simulink model "Test2Part4a"  (R2024a)
settings: Solver=FixedStepAuto  StartTime=0  StopTime=1000  FixedStep=1  MaxStep=1  MinStep=1  RelTol=1e-3
libraries: matrix_library x2
settings Model: NumberOfSteps=1000  Creator=katutu  LastModifiedBy=katutu
settings HardwareCC: ProdBitPerLong=64  ProdHWDeviceType=Intel->x86-64 (Mac OS X)

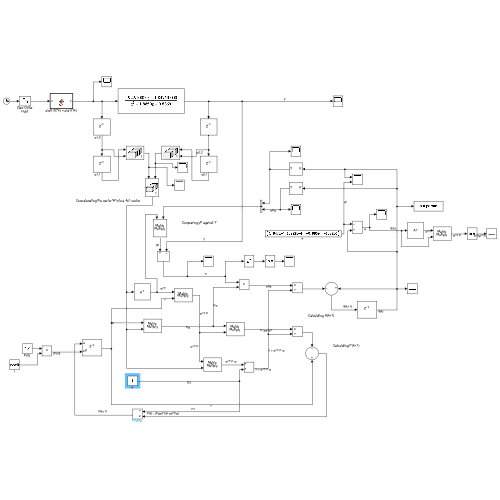
[thumbnail: Simulink's stored preview of the top-level diagram]
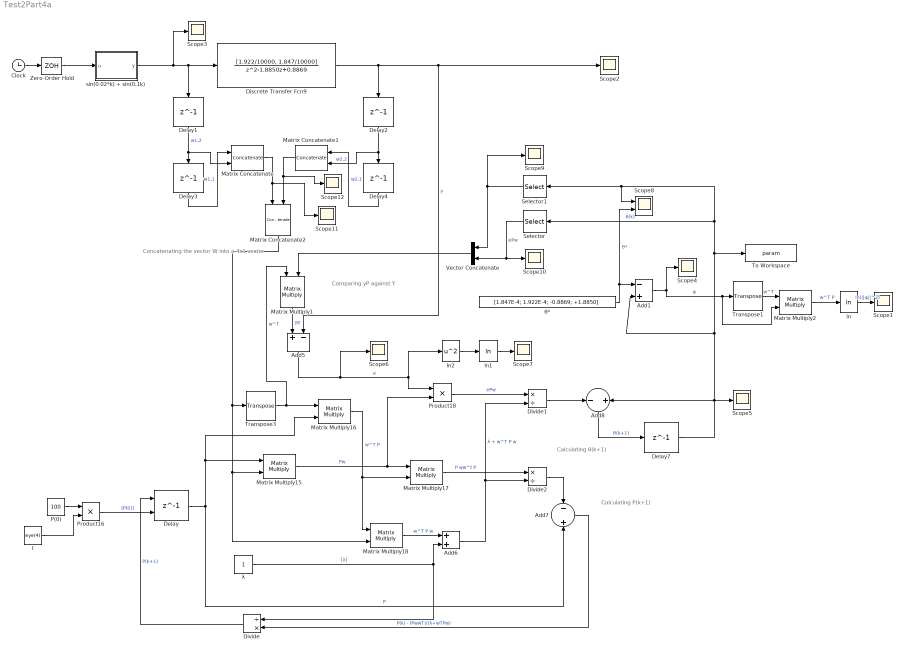
== system Test2Part4a ==
  note: Calculating θ(k+1)
  note: Calculating P(k+1)
  note: Comparing yP against Y
  note: Concatenating the vector W into a 4x1 vector
  Add1 : Sum  Inputs=-+
  Add5 : Sum  Inputs=+-
  Add6 : Sum
  Add7 : Sum  Inputs=-+
  Add8 : Sum  Inputs=-+
  Clock : Clock
  Delay : Delay  DelayLength=1  InitialConditionSource=Input port  InitialCondition=0
      settings: InputPortMap=u0,p4
  Delay{1..4} (4 alike) : Delay  DelayLength=1  InitialCondition=0
  Delay7 : Delay  DelayLength=1  InitialCondition=[0; 0; 0; 0]
  Discrete Transfer Fcn9 : DiscreteTransferFcn  Numerator=[1.922/10000, 1.847/10000]  Denominator=[1 -1.8850 0.8869]
  Divide : Product  Inputs=/*
  Divide1 : Product  Inputs=*/
  Divide2 : Product  Inputs=*/
  I : Constant  Value=eye(4)
  Matrix Concatenate : Concatenate  Mode=Multidimensional array
  Matrix Concatenate1 : Concatenate  Mode=Multidimensional array
  Matrix Concatenate2 : Concatenate  Mode=Multidimensional array
  Matrix Multiply{1..2,15..18} (6 alike) : Product  Multiplication=Matrix(*)
  P(0) : Constant  Value=100
  Product16 : Product
  Product18 : Product
  Scope{1..7,9..12} (11 alike) : Scope
  Scope8 : Scope  NumInputPorts=2
  Selector : Selector  NumberOfDimensions=2  InputPortWidth=3  IndexOptions=Index vector (dialog),Index vector (dialog)  Indices=[3 4],1  OutputSizes=1,1
  Selector1 : Selector  NumberOfDimensions=2  InputPortWidth=3  IndexOptions=Index vector (dialog),Index vector (dialog)  Indices=[1 2],1  OutputSizes=1,1
  To Workspace : ToWorkspace  VariableName=param  SampleTime=-1
      settings: MaxDataPoints=1
  Transpose1 : matrix_library/Transpose
  Transpose3 : matrix_library/Transpose
  Vector Concatenate : Concatenate
  Zero-Order Hold : ZeroOrderHold  SampleTime=-1
  ln : Math  Operator=log
  ln1 : Math  Operator=log
  ln2 : Math  Operator=square
  sin(0.02*k) + sin(0.1k) : MATLAB Function  TreatAsAtomicUnit=on
  θ* : Constant  Value=[1.847E-4; 1.922E-4; -0.8869; +1.8850]
  λ : Constant
  wires:
  Matrix Multiply1/1 -> Add5/1  "yp"
  P(0)/1 -> Product16/1
  Matrix Multiply18/1 -> Add6/1  "w^T P w"
  Transpose3/1 -> Matrix Multiply16/1, Matrix Multiply1/1  "w^T"
  Delay1/1 -> Matrix Concatenate/2, Delay3/1  "w1,2"
  Matrix Multiply15/1 -> Matrix Multiply17/1, Product18/2  "Pw"
  Delay2/1 -> Matrix Concatenate1/2, Delay4/1  "w2,2"
  Delay7/1 -> Scope5/1, Add8/2, Selector/1, Selector1/1, Scope8/1, To Workspace/1, Add1/2  "θ(k)"
  Add6/1 -> Divide2/2, Divide1/2  "λ + w^T P w"
  Product18/1 -> Divide1/1  "ePw"
  Add8/1 -> Delay7/1  "θ(k+1)"
  Delay/1 -> Add7/2, Matrix Multiply15/1, Matrix Multiply16/2  "P"
  Add7/1 -> Divide/2  "P(k) - (PwwT)/(λ+wTPw)"
  I/1 -> Product16/2
  Discrete Transfer Fcn9/1 -> Delay2/1, Scope2/1, Add5/2  "y"
  Product16/1 -> Delay/2  "[P(0)]"
  Delay3/1 -> Matrix Concatenate/1  "w1,1"
  Divide2/1 -> Add7/1
  Matrix Multiply17/1 -> Divide2/1  "P ww^t P"
  Divide1/1 -> Add8/1
  Add5/1 -> Scope6/1, Product18/1, ln2/1  "e"
  λ/1 -> Divide/1, Add6/2  "[λ]"
  Matrix Multiply16/1 -> Matrix Multiply18/1, Matrix Multiply17/2  "w^T P"
  Delay4/1 -> Matrix Concatenate1/1  "w2,1"
  sin(0.02*k) + sin(0.1k)/1(y) -> Scope3/1, Delay1/1, Discrete Transfer Fcn9/1
  θ*/1 -> Add1/1, Scope8/2  "θ*"
  Add1/1 -> Matrix Multiply2/2, Transpose1/1, Scope4/1  "φ"
  ln/1 -> Scope1/1  "ln(||φ||^2)"
  Clock/1 -> Zero-Order Hold/1
  Zero-Order Hold/1 -> sin(0.02*k) + sin(0.1k)/1(u)
  Matrix Concatenate1/1 -> Scope12/1, Matrix Concatenate2/2
  Selector1/1 -> Vector Concatenate/1, Scope9/1
  Matrix Concatenate2/1 -> Matrix Multiply18/2, Matrix Multiply15/2, Transpose3/1
  Matrix Concatenate/1 -> Scope11/1, Matrix Concatenate2/1
  Vector Concatenate/1 -> Matrix Multiply1/2
  Selector/1 -> Scope10/1, Vector Concatenate/2  "ePw"
  ln1/1 -> Scope7/1
  ln2/1 -> ln1/1
  Transpose1/1 -> Matrix Multiply2/1  "w^T"
  Matrix Multiply2/1 -> ln/1  "w^T P"
  Divide/1 -> Delay/1  "P(k+1)"

== matlab function Test2Part4a/sin(0.02*k) + sin(0.1k) ==
  data: u input; y output
function y = fcn(u)


y = sin(0.02*u) + sin(0.1*u);
